simulink model "Ejercicio1BooleanConAnimacion"  (R2024b)
settings: Solver=VariableStepAuto  StartTime=0.0  StopTime=10.0  MaxStep=1e-2  RelTol=1e-5
settings Model: Creator=user  LastModifiedBy=user

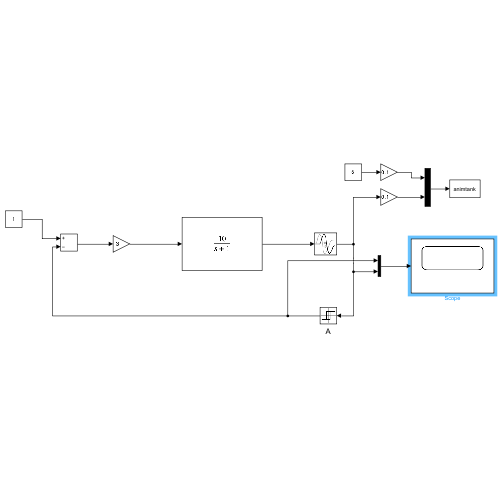
[thumbnail: Simulink's stored preview of the top-level diagram]
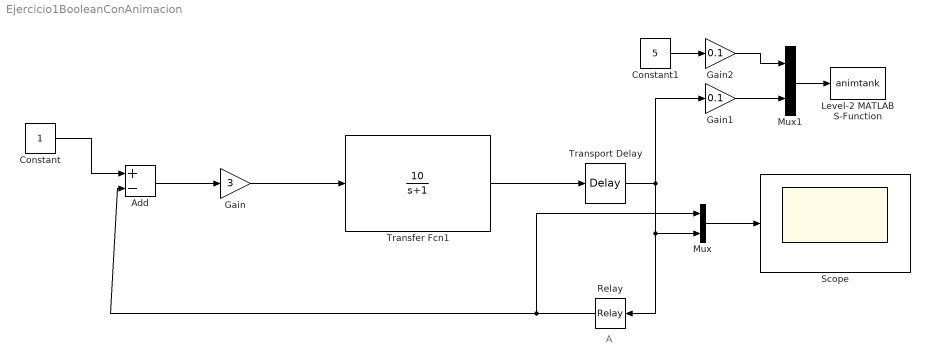
== system Ejercicio1BooleanConAnimacion ==
  note: A
  Add : Sum  Inputs=+-
  Constant : Constant
  Constant1 : Constant  Value=5
  Gain : Gain  Gain=3
  Gain1 : Gain  Gain=0.1
  Gain2 : Gain  Gain=0.1
  Level-2 MATLAB S-Function : M-S-Function  FunctionName=animtank  Parameters=1
  Mux : Mux  Inputs=2
  Mux1 : Mux  Inputs=2
  Relay : Relay  OnSwitchValue=5  OffSwitchValue=5
  Scope : Scope
  Transfer Fcn1 : TransferFcn  Numerator=[10]  Denominator=[1 1]
  Transport Delay : TransportDelay  DelayTime=0.5
  wires:
  Gain/1 -> Transfer Fcn1/1
  Transfer Fcn1/1 -> Transport Delay/1
  Constant/1 -> Add/1
  Relay/1 -> Mux/1, Add/2
  Add/1 -> Gain/1
  Transport Delay/1 -> Mux/2, Relay/1, Gain1/1
  Mux/1 -> Scope/1
  Gain1/1 -> Mux1/2
  Gain2/1 -> Mux1/1
  Mux1/1 -> Level-2 MATLAB S-Function/1
  Constant1/1 -> Gain2/1
